simulink model "EPA_Jumper"  (R2018a)
settings: Solver=FixedStepDiscrete  StartTime=0.0  StopTime=inf  FixedStep=0.001  RelTol=1e-3  EnableMultiTasking=on
model workspace (MAT data in the model file):
  MCOS : class17 (value not decoded)
values from neighbouring files (symbols this model uses):
  bits_current = 12    [Init_EPA_Jumper.m]
  bits_Kd = 12    [Init_EPA_Jumper.m]
  bits_Kp = 12    [Init_EPA_Jumper.m]
  bits_position = 16    [Init_EPA_Jumper.m]
  bits_velocity = 12    [Init_EPA_Jumper.m]
  KD_MAX = 5.0    (= 5)    [Init_EPA_Jumper.m]
  KD_MIN = 0.0    (= 0)    [Init_EPA_Jumper.m]
  KP_MAX = 500.0    (= 500)    [Init_EPA_Jumper.m]
  KP_MIN = 0.0    (= 0)    [Init_EPA_Jumper.m]
  P_MAX = 95.5    [Init_EPA_Jumper.m]
  P_MIN = -95.5    [Init_EPA_Jumper.m]
  PressureFilter_CutOffFreq = 20    [Init_EPA_Jumper.m]
  PressureFilter_Gain = 1    [Init_EPA_Jumper.m]
  ReadingVoltage = 5    [Init_EPA_Jumper.m]
  T_MAX = 18.0    (= 18)    [Init_EPA_Jumper.m]
  T_MIN = -18.0    (= -18)    [Init_EPA_Jumper.m]
  V_MAX = 45.0    (= 45)    [Init_EPA_Jumper.m]
  V_MIN = -45.0    (= -45)    [Init_EPA_Jumper.m]
  voltageBias = -2.5    [Init_EPA_Jumper.m]
  voltageMultiplier = 2.5    [Init_EPA_Jumper.m]
  VoltageResolution = 1023.0    (= 1023)    [Init_EPA_Jumper.m]
libraries: xpcethercatlib x76, slrtlib x15, simulink x10, peGeneralControl x9
(part 3 of 3)

== matlab function EPA_Jumper/Ethernet Communication/Inputs/PAMs Slave/MATLAB Function ==
  data: sensorValue input; pressure output; voltageMultiplier parameter; voltageBias parameter; ReadingVoltage parameter; VoltageResolution parameter
function pressure   = fcn(sensorValue,voltageMultiplier, voltageBias,ReadingVoltage, VoltageResolution)
pressure   = PressureSensor(sensorValue,voltageMultiplier, voltageBias,ReadingVoltage,VoltageResolution);
end

== matlab function EPA_Jumper/Ethernet Communication/Inputs/PAMs Slave/MATLAB Function1 ==
  data: sensorValue input; pressure output; voltageMultiplier parameter; voltageBias parameter; ReadingVoltage parameter; VoltageResolution parameter
function pressure   = fcn(sensorValue,voltageMultiplier, voltageBias,ReadingVoltage, VoltageResolution)
pressure   = PressureSensor(sensorValue,voltageMultiplier, voltageBias,ReadingVoltage,VoltageResolution);
end

== matlab function EPA_Jumper/Ethernet Communication/Inputs/PAMs Slave/MATLAB Function2 ==
  data: sensorValue input; pressure output; voltageMultiplier parameter; voltageBias parameter; ReadingVoltage parameter; VoltageResolution parameter
function pressure   = fcn(sensorValue,voltageMultiplier, voltageBias,ReadingVoltage, VoltageResolution)
pressure   = PressureSensor(sensorValue,voltageMultiplier, voltageBias,ReadingVoltage,VoltageResolution);
end

== matlab function EPA_Jumper/Ethernet Communication/Inputs/PAMs Slave/MATLAB Function3 ==
  data: sensorValue input; pressure output; voltageMultiplier parameter; voltageBias parameter; ReadingVoltage parameter; VoltageResolution parameter
function pressure   = fcn(sensorValue,voltageMultiplier, voltageBias,ReadingVoltage, VoltageResolution)
pressure   = PressureSensor(sensorValue,voltageMultiplier, voltageBias,ReadingVoltage,VoltageResolution);
end

== matlab function EPA_Jumper/Ethernet Communication/Inputs/PAMs Slave/MATLAB Function4 ==
  data: sensorValue input; pressure output; voltageMultiplier parameter; voltageBias parameter; ReadingVoltage parameter; VoltageResolution parameter
function pressure   = fcn(sensorValue,voltageMultiplier, voltageBias,ReadingVoltage, VoltageResolution)
pressure   = PressureSensor(sensorValue,voltageMultiplier, voltageBias,ReadingVoltage,VoltageResolution);
end

== matlab function EPA_Jumper/Ethernet Communication/Inputs/PAMs Slave/MATLAB Function5 ==
  data: sensorValue input; pressure output; voltageMultiplier parameter; voltageBias parameter; ReadingVoltage parameter; VoltageResolution parameter
function pressure   = fcn(sensorValue,voltageMultiplier, voltageBias,ReadingVoltage, VoltageResolution)
pressure   = PressureSensor(sensorValue,voltageMultiplier, voltageBias,ReadingVoltage,VoltageResolution);
end

== matlab function EPA_Jumper/Ethernet Communication/Inputs/PAMs Slave/MATLAB Function6 ==
  data: sensorValue input; pressure output; voltageMultiplier parameter; voltageBias parameter; ReadingVoltage parameter; VoltageResolution parameter
function pressure   = fcn(sensorValue,voltageMultiplier, voltageBias,ReadingVoltage, VoltageResolution)
pressure   = PressureSensor(sensorValue,voltageMultiplier, voltageBias,ReadingVoltage,VoltageResolution);
end

== matlab function EPA_Jumper/Ethernet Communication/Inputs/PAMs Slave/MATLAB Function7 ==
  data: sensorValue input; pressure output; voltageMultiplier parameter; voltageBias parameter; ReadingVoltage parameter; VoltageResolution parameter
function pressure   = fcn(sensorValue,voltageMultiplier, voltageBias,ReadingVoltage, VoltageResolution)
pressure   = PressureSensor(sensorValue,voltageMultiplier, voltageBias,ReadingVoltage,VoltageResolution);
end

== matlab function EPA_Jumper/Ethernet Communication/Inputs/PAMs Slave/MATLAB Function8 ==
  data: sensorValue input; pressure output; voltageMultiplier parameter; voltageBias parameter; ReadingVoltage parameter; VoltageResolution parameter
function pressure   = fcn(sensorValue,voltageMultiplier, voltageBias,ReadingVoltage, VoltageResolution)
pressure   = PressureSensor(sensorValue,voltageMultiplier, voltageBias,ReadingVoltage,VoltageResolution);
end

== matlab function EPA_Jumper/PAMs/PAM_1/Solenoids ==
  data: control input; intake output; inside_deadzone input; outtake output; inside_deadzone_1 output; deadzone_in input; deadzone_out input; PAMs_on input; System_on input
function [intake, outtake,inside_deadzone_1] = fcn(control, inside_deadzone, deadzone_in, deadzone_out,PAMs_on,System_on)

[intake, outtake,inside_deadzone_1] = Solenoid(control, inside_deadzone, deadzone_in, deadzone_out,PAMs_on,System_on);
    
  
end

== matlab function EPA_Jumper/PAMs/PAM_2/Solenoids ==
  data: control input; intake output; inside_deadzone input; outtake output; inside_deadzone_1 output; deadzone_in input; deadzone_out input; PAMs_on input; System_on input
function [intake, outtake,inside_deadzone_1] = fcn(control, inside_deadzone, deadzone_in, deadzone_out,PAMs_on,System_on)

[intake, outtake,inside_deadzone_1] = Solenoid(control, inside_deadzone, deadzone_in, deadzone_out,PAMs_on,System_on);
    
  
end

== matlab function EPA_Jumper/PAMs/PAM_3/Solenoids ==
  data: control input; intake output; inside_deadzone input; outtake output; inside_deadzone_1 output; deadzone_in input; deadzone_out input; PAMs_on input; System_on input
function [intake, outtake,inside_deadzone_1] = fcn(control, inside_deadzone, deadzone_in, deadzone_out,PAMs_on,System_on)

[intake, outtake,inside_deadzone_1] = Solenoid(control, inside_deadzone, deadzone_in, deadzone_out,PAMs_on,System_on);
    
  
end

== matlab function EPA_Jumper/PAMs/PAM_4/Solenoids ==
  data: control input; intake output; inside_deadzone input; outtake output; inside_deadzone_1 output; deadzone_in input; deadzone_out input; PAMs_on input; System_on input
function [intake, outtake,inside_deadzone_1] = fcn(control, inside_deadzone, deadzone_in, deadzone_out,PAMs_on,System_on)

[intake, outtake,inside_deadzone_1] = Solenoid(control, inside_deadzone, deadzone_in, deadzone_out,PAMs_on,System_on);
    
  
end

== matlab function EPA_Jumper/PAMs/PAM_5/Solenoids ==
  data: control input; intake output; inside_deadzone input; outtake output; inside_deadzone_1 output; deadzone_in input; deadzone_out input; PAMs_on input; System_on input
function [intake, outtake,inside_deadzone_1] = fcn(control, inside_deadzone, deadzone_in, deadzone_out,PAMs_on,System_on)

[intake, outtake,inside_deadzone_1] = Solenoid(control, inside_deadzone, deadzone_in, deadzone_out,PAMs_on,System_on);
    
  
end

== matlab function EPA_Jumper/PAMs/PAM_6/Solenoids ==
  data: control input; intake output; inside_deadzone input; outtake output; inside_deadzone_1 output; deadzone_in input; deadzone_out input; PAMs_on input; System_on input
function [intake, outtake,inside_deadzone_1] = fcn(control, inside_deadzone, deadzone_in, deadzone_out,PAMs_on,System_on)

[intake, outtake,inside_deadzone_1] = Solenoid(control, inside_deadzone, deadzone_in, deadzone_out,PAMs_on,System_on);
    
  
end

== matlab function EPA_Jumper/PAMs/PAM_7/Solenoids ==
  data: control input; intake output; inside_deadzone input; outtake output; inside_deadzone_1 output; deadzone_in input; deadzone_out input; PAMs_on input; System_on input
function [intake, outtake,inside_deadzone_1] = fcn(control, inside_deadzone, deadzone_in, deadzone_out,PAMs_on,System_on)

[intake, outtake,inside_deadzone_1] = Solenoid(control, inside_deadzone, deadzone_in, deadzone_out,PAMs_on,System_on);
    
  
end

== matlab function EPA_Jumper/PAMs/PAM_8/Solenoids ==
  data: control input; intake output; inside_deadzone input; outtake output; inside_deadzone_1 output; deadzone_in input; deadzone_out input; PAMs_on input; System_on input
function [intake, outtake,inside_deadzone_1] = fcn(control, inside_deadzone, deadzone_in, deadzone_out,PAMs_on,System_on)

[intake, outtake,inside_deadzone_1] = Solenoid(control, inside_deadzone, deadzone_in, deadzone_out,PAMs_on,System_on);
    
  
end

== matlab function EPA_Jumper/PAMs/PAM_9/Solenoids ==
  data: control input; intake output; inside_deadzone input; outtake output; inside_deadzone_1 output; deadzone_in input; deadzone_out input; PAMs_on input; System_on input
function [intake, outtake,inside_deadzone_1] = fcn(control, inside_deadzone, deadzone_in, deadzone_out,PAMs_on,System_on)

[intake, outtake,inside_deadzone_1] = Solenoid(control, inside_deadzone, deadzone_in, deadzone_out,PAMs_on,System_on);
    
  
end

== matlab function EPA_Jumper/GRF/GRFz/COP ==
  data: grf1 input; xPosition output; grf2 input; yPosition output; grf3 input; grf4 input
function [xPosition, yPosition] = fcn(grf1, grf2, grf3, grf4)
    % Sensor positions
    p1 = [52, 42];
    p2 = [52, 0];
    p3 = [0, 0];
    p4 = [0, 42];
    
    % Calculate total force
    F_total = grf1 + grf2 + grf3 + grf4;
    
    % Calculate moments
    M_x = grf1 * p1(1) + grf2 * p2(1) + grf3 * p3(1) + grf4 * p4(1);
    M_y = grf1 * p1(2) + grf2 * p2(2) + grf3 * p3(2) + grf4 * p4(2);
    
    % Calculate center of pressure
    xPosition = M_y / F_total;
    yPosition = M_x / F_total;
end
